simulink model "hustemp"  (R2017b)
settings: Solver=ode45  StartTime=0.0  StopTime=31536000  FixedStep=100  MinStep=100  RelTol=1e-3  AbsTol=1e-6
PreLoadFcn:
  | thermdat
values from neighbouring files (symbols this model uses):
  Ct = 1800000    [husdata.mat]
  dt = 1    [husdata.mat]
  Rt = 0.0045    [husdata.mat]
settings Model: ExtModeTrigMode=oneshot  ExtModeArmWhenConnect=off  ExtModeAutoUpdateStatusClock=off  Creator=nikita  LastModifiedBy=Morten
settings DataIOCC: ExternalInput=[]  InitialState=[]  SaveFormat=Array  SignalLoggingSaveFormat=ModelDataLogs  SaveOutput=off  SaveTime=off  SignalLoggingName=sigsOut
settings OptimizationCC: BlockReduction=off  BooleanDataType=off
settings DebuggingCC: SaveWithParameterizedLinksMsg=none  UnderspecifiedInitializationDetection=Classic  MergeDetectMultiDrivingBlocksExec=none  SignalResolutionControl=TryResolveAllWithWarning  MultiTaskDSMMsg=warning  MultiTaskCondExecSysMsg=none  IntegerOverflowMsg=none
settings HardwareCC: ProdBitPerPointer=32  ProdBitPerSizeT=32  ProdBitPerPtrDiffT=32  ProdLargestAtomicFloat=None  ProdIntDivRoundTo=Undefined  ProdEndianess=Unspecified  ProdWordSize=32  ProdHWDeviceType=32-bit Generic  TargetUnknown=on
settings ModelReferenceCC: PropagateSignalLabelsOutOfModel=off
settings GRTTargetCC: TargetFcnLib=ansi_tfl_tmw.mat  TargetLangStandard=C89/C90 (ANSI)  CodeReplacementLibrary=ANSI_C  MultiwordLength=256  ModelReferenceCompliant=off  CompOptLevelCompliant=off  CombineOutputUpdateFcns=off  MatFileLogging=off  CPPClassGenCompliant=off  GRTInterface=on
settings ConfigComp: CovMetricSettings=dw  CovHtmlReporting=on  CovSaveCumulativeToWorkspaceVar=on  CovSaveSingleToWorkspaceVar=on  CovExternalEMLEnable=off

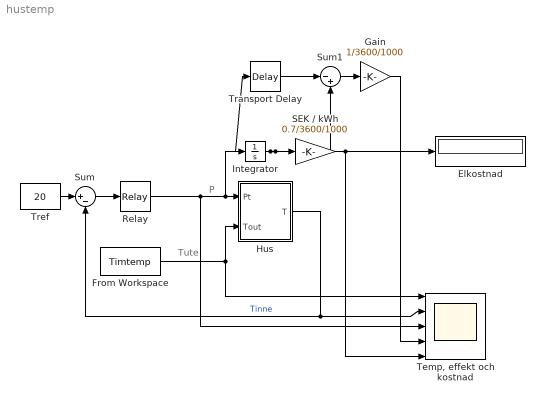
== system hustemp ==
  note: Tute
  note: P
  Elkostnad : Display
  From Workspace : FromWorkspace  VariableName=Timtemp  SampleTime=3600
  Gain : Gain  Gain=1/3600/1000  SaturateOnIntegerOverflow=on  OutDataTypeStr=Inherit: Same as input  ParamDataTypeStr=Inherit: Same as input
  Hus : Subsystem
      mask Display: plot(0,0,100,100,[20,80,80,20,20],[20,20,70,70,20],[15,50,85,15],[70,90,70,70],[42,42,29,29],[20,44,44,20],[52,68,68,52,52],[55,55,44,44,55])
  Integrator : Integrator
  Relay : Relay  OnSwitchValue=dt/2  OffSwitchValue=-dt/2  OnOutputValue=Pt
  SEK / kWh : Gain  Gain=0.7/3600/1000  SaturateOnIntegerOverflow=on  OutDataTypeStr=Inherit: Same as input  ParamDataTypeStr=Inherit: Same as input
  Sum : Sum  Inputs=|+-  SaturateOnIntegerOverflow=on
  Sum1 : Sum  Inputs=|-+  SaturateOnIntegerOverflow=on
  "Temp, effekt och kostnad" : Scope  NumInputPorts=5
  Transport Delay : TransportDelay  DelayTime=3600
  Tref : Constant  Value=20
  wires:
  Integrator/1 -> SEK / kWh/1, Sum1/2, Transport Delay/1
  Hus/1(T) -> "Temp, effekt och kostnad"/2, Sum/2  "Tinne"
  SEK / kWh/1 -> Elkostnad/1, "Temp, effekt och kostnad"/5
  From Workspace/1 -> "Temp, effekt och kostnad"/1, Hus/2(Tout)
  Relay/1 -> Hus/1(Pt), Integrator/1, "Temp, effekt och kostnad"/3
  Tref/1 -> Sum/1
  Sum/1 -> Relay/1
  Transport Delay/1 -> Sum1/1
  Sum1/1 -> Gain/1
  Gain/1 -> "Temp, effekt och kostnad"/4

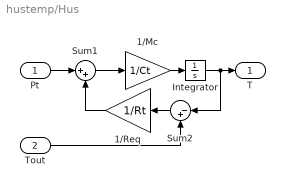
== system hustemp/Hus ==
  Pt : Inport
  Tout : Inport  Port=2
  1/Mc : Gain  Gain=1/Ct  SaturateOnIntegerOverflow=on  OutDataTypeStr=Inherit: Same as input  ParamDataTypeStr=Inherit: Same as input
  1/Req : Gain  Gain=1/Rt  SaturateOnIntegerOverflow=on  OutDataTypeStr=Inherit: Same as input  ParamDataTypeStr=Inherit: Same as input
  Integrator : Integrator  InitialCondition=22
  Sum1 : Sum  Inputs=|++  SaturateOnIntegerOverflow=on  InputSameDT=on  OutDataTypeStr=Inherit: Same as first input
  Sum2 : Sum  Inputs=|-+  SaturateOnIntegerOverflow=on  InputSameDT=on  OutDataTypeStr=Inherit: Same as first input
  T : Outport  InitialOutput=0
  wires:
  Tout/1 -> Sum2/2
  Pt/1 -> Sum1/1
  Sum1/1 -> 1/Mc/1
  Sum2/1 -> 1/Req/1
  1/Req/1 -> Sum1/2
  1/Mc/1 -> Integrator/1
  Integrator/1 -> Sum2/1, T/1
